simulink model "cxema"  (R2015b)
settings: Solver=VariableStepAuto  StartTime=0.0  StopTime=10.0  RelTol=1e-3
settings Model: Creator=hohotulca  LastModifiedBy=hohotulca

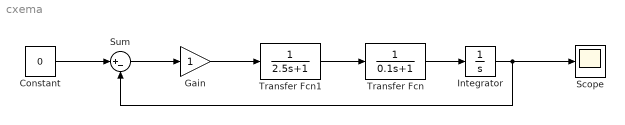
== system cxema ==
  Constant : Constant  Value=0
  Gain : Gain
  Integrator : Integrator
  Scope : Scope
  Sum : Sum  Inputs=|+-
  Transfer Fcn : TransferFcn  Denominator=[0.1 1]
  Transfer Fcn1 : TransferFcn  Denominator=[2.5 1]
  wires:
  Transfer Fcn/1 -> Integrator/1
  Sum/1 -> Gain/1
  Gain/1 -> Transfer Fcn1/1
  Transfer Fcn1/1 -> Transfer Fcn/1
  Integrator/1 -> Scope/1, Sum/2
  Constant/1 -> Sum/1
